simulink model "lab3c"  (R2022b)
settings: Solver=FixedStepAuto  StartTime=0.0  StopTime=1.0  FixedStep=1/1024  RelTol=1e-3
values from neighbouring files (symbols this model uses):
  amp = i    [lab3a.m]    (also in lab3a_script.m = db2mag(cur_pow); lab3bscript.m)
  ex_r2r = r2r(N, 0.02*i)    [lab3a_script.m]
  N = 10    [lab3a_script.m]
settings Model: Creator=simja  LastModifiedBy=simja
settings DataIOCC: ReturnWorkspaceOutputs=off

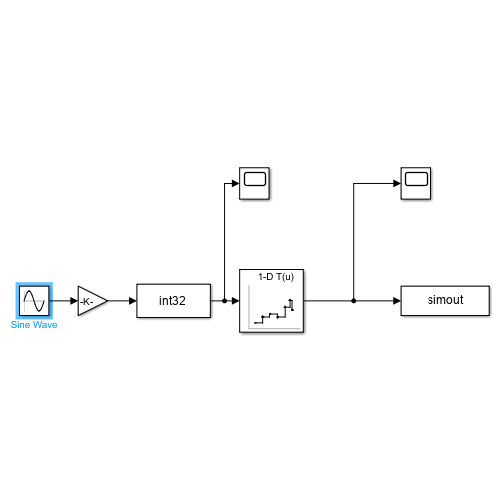
[thumbnail: Simulink's stored preview of the top-level diagram]
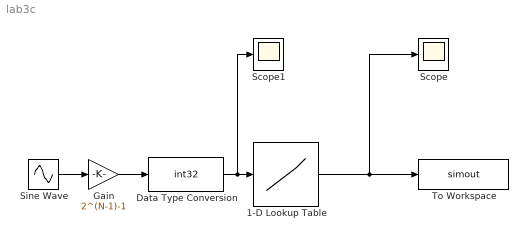
== system lab3c ==
  1-D Lookup Table : Lookup_n-D  NumberOfTableDimensions=1  BreakpointsForDimension1=-2^(N-1):(2^(N-1))-1  Table=ex_r2r  InterpMethod=Flat  InternalRulePriority=Speed  OutDataTypeStr=double  RndMeth=Simplest
  Data Type Conversion : DataTypeConversion  OutDataTypeStr=int32  RndMeth=Nearest  SaturateOnIntegerOverflow=off
  Gain : Gain  Gain=2^(N-1)-1
  Scope : Scope
  Scope1 : Scope
  Sine Wave : Sin  Amplitude=amp  Frequency=2*5*pi  SampleTime=0
  To Workspace : ToWorkspace  VariableName=simout  SaveFormat=Structure With Time  SampleTime=-1
  wires:
  1-D Lookup Table/1 -> Scope/1, To Workspace/1
  Data Type Conversion/1 -> Scope1/1, 1-D Lookup Table/1
  Gain/1 -> Data Type Conversion/1
  Sine Wave/1 -> Gain/1
